simulink model "Maglev_Hardware_24a_R4"  (R2024a)
settings: Solver=ode3  StartTime=0.0  StopTime=inf  FixedStep=.001  RelTol=1e-3  EnableMultiTasking=on
libraries: arduinolib x5, simulink x1
settings Model: ModifiedByFormat=C. Gokcek  ExtModeTrigDuration=2  Creator=C. Gokcek  LastModifiedBy=C. Gokcek
settings SolverCC: AlgebraicLoopSolver=TrustRegion
settings DataIOCC: LimitDataPoints=on  SaveFormat=Array  ReturnWorkspaceOutputs=off
settings OptimizationCC: EnhancedBackFolding=on  PassReuseOutputArgsThreshold=0  MaxStackSize=64  OptimizeBlockOrder=speed  DifferentSizesBufferReuse=on  OptimizationCustomize=off
settings DebuggingCC: UnderspecifiedInitializationDetection=Classic  MergeDetectMultiDrivingBlocksExec=none  ParameterTunabilityLossMsg=error  UnconnectedInputMsg=warning  UnconnectedOutputMsg=warning  UnconnectedLineMsg=warning  StateNameClashWarn=warning  SFUnexpectedBacktrackingDiag=warning  SFNoUnconditionalDefaultTransitionDiag=warning  SFExecutionAtInitializationDiag=none  ArithmeticOperatorsInVariantConditions=warning
settings HardwareCC: ProdBitPerInt=16  ProdBitPerPointer=16  ProdBitPerSizeT=16  ProdBitPerPtrDiffT=16  ProdLargestAtomicFloat=None  ProdWordSize=8  ProdHWDeviceType=Atmel->AVR  UseEmbeddedCoderFeatures=off  UseSimulinkCoderFeatures=off
settings ModelReferenceCC: EnableRefExpFcnMdlSchedulingChecks=on  PropagateSignalLabelsOutOfModel=off
settings SFSimCC: SimUseLocalCustomCode=off  MATLABDynamicMemAlloc=off  CustomCodeUndefinedFunction=UseInterfaceOnly
settings RTWCC: Description=Embedded Coder  SystemTargetFile=ert.tlc  HardwareBoard=Arduino Mega 2560  TemplateMakefile=ert_default_tmf  RTWVerbose=off  RTWUseLocalCustomCode=off  Toolchain=Arduino AVR  BuildConfiguration=Faster Runs  GPUComputeCapability=3.5
settings CodeAppCC: ForceParamTrailComments=on  OperatorAnnotations=on
settings ERTTargetCC: ERTCustomFileBanners=off  SupportContinuousTime=on  SupportNonInlinedSFcns=on  RemoveResetFunc=off  SupportVariableSizeSignals=on  ModelStepFunctionPrototypeControlCompliant=off  ExtModeTransport=3  ExtModeStaticAlloc=on  ExtModeStaticAllocSize=2048  ExtModeMexFile=ext_xcp  ExtModeIntrfLevel=Level2 - Open
settings ConfigComp: CovMetricSettings=dw  CovSaveCumulativeToWorkspaceVar=on  CovSaveSingleToWorkspaceVar=on  CovExternalEMLEnable=off

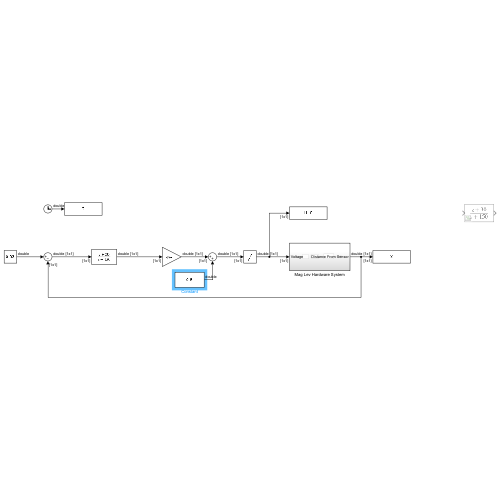
[thumbnail: Simulink's stored preview of the top-level diagram]
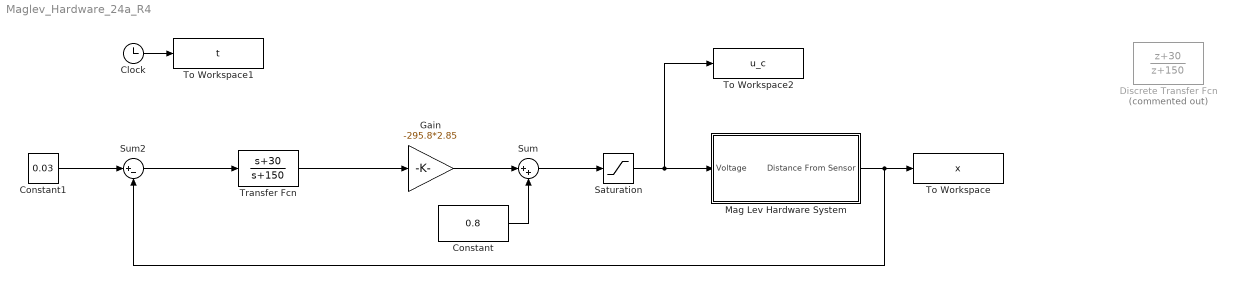
== system Maglev_Hardware_24a_R4 ==
  Clock : Clock
  Constant : Constant  Value=0.8
  Constant1 : Constant  Value=0.03
  Discrete Transfer Fcn : DiscreteTransferFcn  Commented=on  Numerator=[1 30]  Denominator=[1 150]
  Gain : Gain  Gain=-295.8*2.85
  Mag Lev Hardware System : Subsystem
  Saturation : Saturate  UpperLimit=3.25  LowerLimit=-3.25
  Sum : Sum  Inputs=|++
  Sum2 : Sum  Inputs=|+-
  To Workspace : ToWorkspace  VariableName=x  SampleTime=-1
      settings: Save2DSignal=2-D array (concatenate along first dimension)
  To Workspace1 : ToWorkspace  VariableName=t  SampleTime=-1
      settings: Save2DSignal=2-D array (concatenate along first dimension)
  To Workspace2 : ToWorkspace  VariableName=u_c  SampleTime=-1
      settings: Save2DSignal=2-D array (concatenate along first dimension)
  Transfer Fcn : TransferFcn  Numerator=[1 30]  Denominator=[1 150]
  wires:
  Clock/1 -> To Workspace1/1
  Constant1/1 -> Sum2/1
  Gain/1 -> Sum/1
  Constant/1 -> Sum/2
  Sum/1 -> Saturation/1
  Saturation/1 -> Mag Lev Hardware System/1(Voltage), To Workspace2/1
  Mag Lev Hardware System/1(Distance From Sensor) -> Sum2/2, To Workspace/1
  Sum2/1 -> Transfer Fcn/1
  Transfer Fcn/1 -> Gain/1

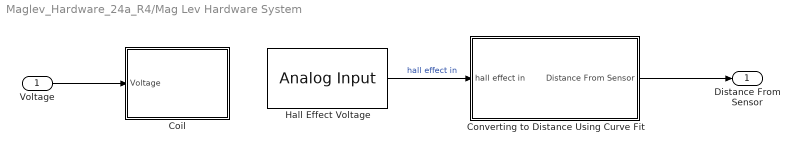
== system Maglev_Hardware_24a_R4/Mag Lev Hardware System ==
  Voltage : Inport
  Coil : Subsystem
  Converting to Distance Using Curve Fit : Subsystem
  Hall Effect Voltage : arduinolib/Analog Input  pinNumber=3  ReadResultsOnly=off  ConversionTriggerSource=Software  ExternalTriggerType=uint32( 0 )  OutputDataType=uint16  EnableConversionCompleteNotify=off  EnableOuputStatus=off  SampleTime=-1  blockPlatform=arduino
  Distance From Sensor : Outport
  wires:
  Voltage/1 -> Coil/1(Voltage)
  Hall Effect Voltage/1 -> Converting to Distance Using Curve Fit/1(hall effect in)  "hall effect in"
  Converting to Distance Using Curve Fit/1(Distance From Sensor) -> Distance From Sensor/1

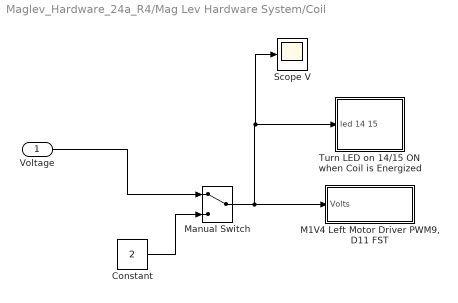
== system Maglev_Hardware_24a_R4/Mag Lev Hardware System/Coil ==
  Voltage : Inport
  Constant : Constant  Value=2
  "M1V4 Left Motor Driver PWM9, D11 FST" : Subsystem  mask(Motor Driver){Vsupply=3.25}
      mask prompts: Vsupply "Driver Voltage"
      mask help:
      | Use a single PWM and a single Digtial out to control the magnitude and direction of a motor
      |
      | Specify driver supply voltage (3.25 for USB with SN754410)
      |
      | Driver supply voltage can be measured direcly by turning the motor fully on (100% duty cycle) and measuring the voltage across the motor leads.  This is the maximum voltage available to the motor and is used to scale from volts to PWM value 0-255.
      |
      | Note this value must be changed if the supply voltage to the driver is changed, for example, by using batteries.
      |
      | Vsupply is the maximum voltage your system is capable of supplying to system given the power supply. It needs to be measured depending on the power supply.
      mask Display:
      | port_label('input',1,'Volts')
      | text(15,5,['Vsupply=' num2str(Vsupply)])
  Manual Switch : ManualSwitch
  Scope V : Scope
  Turn LED on 14/15 ON when Coil is Energized : Subsystem
  wires:
  Manual Switch/1 -> Scope V/1, Turn LED on 14/15 ON when Coil is Energized/1(led 14 15), "M1V4 Left Motor Driver PWM9, D11 FST"/1(Volts)
  Constant/1 -> Manual Switch/2
  Voltage/1 -> Manual Switch/1

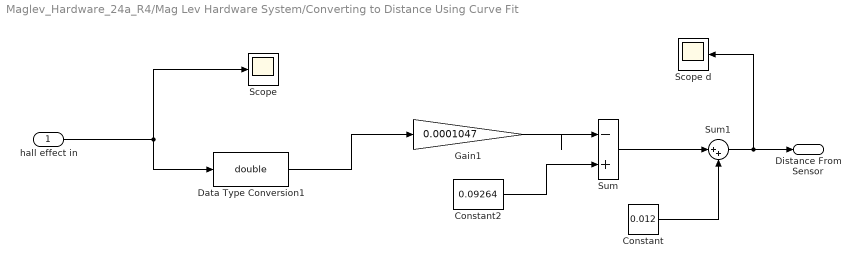
== system Maglev_Hardware_24a_R4/Mag Lev Hardware System/Converting to Distance Using Curve Fit ==
  hall effect in : Inport
  Constant : Constant  Value=0.012
  Constant2 : Constant  Value=0.09264
  Data Type Conversion1 : DataTypeConversion  OutDataTypeStr=double  SaturateOnIntegerOverflow=off  RndMeth=Floor
  Gain1 : Gain  Gain=0.0001047
  Scope : Scope
  Scope d : Scope
  Sum : Sum  Inputs=|-+
  Sum1 : Sum  Inputs=|++
  Distance From Sensor : Outport
  wires:
  hall effect in/1 -> Data Type Conversion1/1, Scope/1
  Data Type Conversion1/1 -> Gain1/1
  Constant/1 -> Sum1/2
  Sum/1 -> Sum1/1
  Constant2/1 -> Sum/2
  Sum1/1 -> Scope d/1, Distance From Sensor/1
  Gain1/1 -> Sum/1

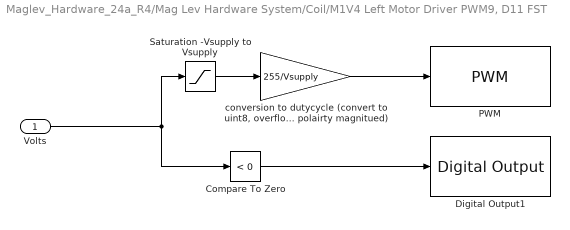
== system Maglev_Hardware_24a_R4/Mag Lev Hardware System/Coil/M1V4 Left Motor Driver PWM9, D11 FST ==
  Volts : Inport
  Compare To Zero : simulink/Logic and Bit Operations/Compare To Zero  relop=<  OutDataTypeStr=boolean
  Digital Output1 : arduinolib/Digital Output  pinNumber=11  Direction=output  blockPlatform=arduino
  PWM : arduinolib/PWM  pinNumber=9  frequencyType=Default  desiredFrequency=490.2  achievableFrequency=490.2
  Saturation -Vsupply to Vsupply : Saturate  UpperLimit=Vsupply  LowerLimit=-Vsupply  OutDataTypeStr=single
  "conversion to dutycycle (convert to uint8, overflow will provide reverse polairty magnitued)" : Gain  Gain=255/Vsupply  OutDataTypeStr=uint8
  wires:
  Volts/1 -> Compare To Zero/1, Saturation -Vsupply to Vsupply/1
  Saturation -Vsupply to Vsupply/1 -> "conversion to dutycycle (convert to uint8, overflow will provide reverse polairty magnitued)"/1
  "conversion to dutycycle (convert to uint8, overflow will provide reverse polairty magnitued)"/1 -> PWM/1
  Compare To Zero/1 -> Digital Output1/1

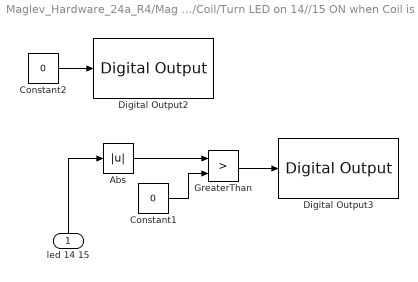
== system Maglev_Hardware_24a_R4/Mag Lev Hardware System/Coil/Turn LED on 14//15 ON when Coil is Energized ==
  led 14 15 : Inport
  Abs : Abs  SaturateOnIntegerOverflow=off
  Constant1 : Constant  Value=0  OutDataTypeStr=boolean  SampleTime=0
  Constant2 : Constant  Value=0  OutDataTypeStr=boolean  SampleTime=0
  Digital Output2 : arduinolib/Digital Output  pinNumber=14  Direction=output  blockPlatform=arduino
  Digital Output3 : arduinolib/Digital Output  pinNumber=15  Direction=output  blockPlatform=arduino
  GreaterThan : RelationalOperator  Operator=>  OutDataTypeStr=boolean  RndMeth=Simplest  InputSameDT=off
  wires:
  Constant2/1 -> Digital Output2/1
  led 14 15/1 -> Abs/1
  Abs/1 -> GreaterThan/1
  Constant1/1 -> GreaterThan/2
  GreaterThan/1 -> Digital Output3/1
